simulink model "adcddcxaui_pass15"  (Simulink 6.2)
settings: Solver=ode45  StartTime=0.0  StopTime=100  RelTol=1e-3
undefined symbols (not defined in the file): BitWidth
libraries: xbsIndex_r3 x402, casper_library x31, xps_library x31
(part 1 of 5)
settings Model: LastModifiedBy=lspitler
settings DebuggingCC: SolverPrmCheckMsg=warning

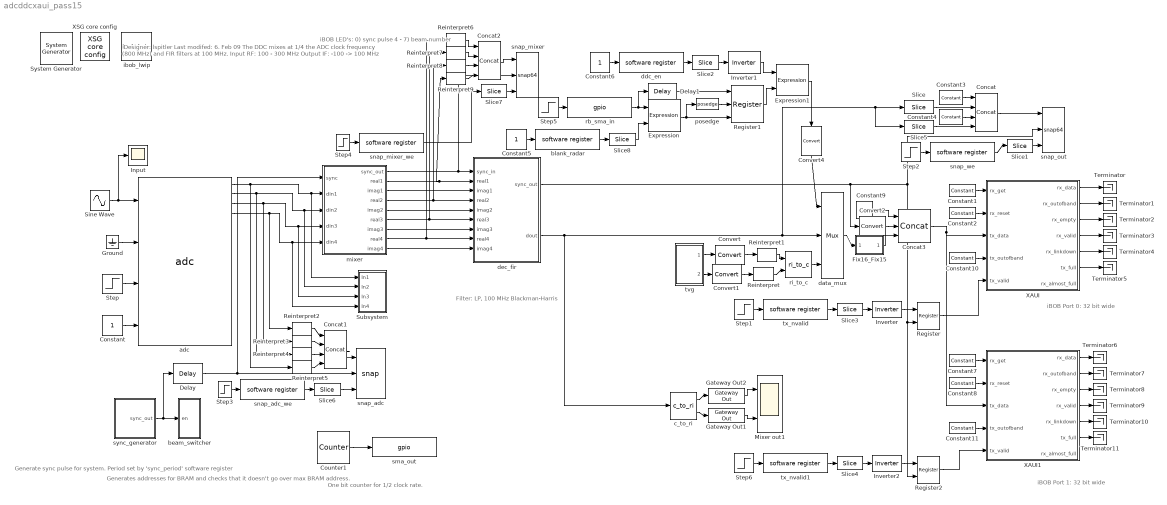
== system adcddcxaui_pass15 ==
  note: Designer: lspitler
      | Last modifed: 6. Feb 09
      | The DDC mixes at 1/4 the ADC clock frequency (800 MHz)
      | and FIR filters at 100 MHz.
      | Input RF: 100 - 300 MHz
      | Output IF: -100 -> 100 MHz
  note: Filter:
      | LP, 100 MHz Blackman-Harris
  note: iBOB Port 0: 32 bit wide
  note: One bit counter
      | for 1/2 clock rate.
  note: Generate sync pulse for system.
      | Period set by 'sync_period'
      | software register
  note: iBOB LED's:
      | 0) sync pulse
      | 4 - 7) beam number
  note: Generates addresses
      | for BRAM and checks
      | that it doesn't go over
      | max BRAM address.
  note: iBOB Port 1: 32 bit wide
  " System Generator" : xbsIndex_r3/ System Generator  Tag=genX  xilinxfamily=Virtex2P  part=xc2vp50  speed=-7  package=ff1152  synthesis_tool=XST  directory=./adcddcxaui_pass/sysgen  testbench=off  simulink_period=1  sysclk_period=5  incr_netlist=off  trim_vbits=Everywhere in SubSystem  dbl_ovrd=According to Block Masks  core_generation=According to Block Masks  run_coregen=off  deprecated_control=off  eval_field=0
      settings: AttributesFormatString=System\nGenerator
  Concat : xbsIndex_r3/Concat  num_inputs=4  explicit_period=on  period=1  dbl_ovrd=off
  Concat1 : xbsIndex_r3/Concat  num_inputs=4  explicit_period=on  period=1  dbl_ovrd=off
  Concat2 : xbsIndex_r3/Concat  num_inputs=4  explicit_period=on  period=1  dbl_ovrd=off
  Concat3 : xbsIndex_r3/Concat  num_inputs=3  explicit_period=on  period=1  dbl_ovrd=off
  Constant : Constant
  Constant1 : xbsIndex_r3/Constant  const=1  equ=P=C  arith_type=Boolean  n_bits=1  bin_pt=0  opselect=C  inp2=PCIN>>17  opr=+  inp1=P  carry=CIN  iostate=0  explicit_period=on  period=1  dbl_ovrd=off
  Constant10 : xbsIndex_r3/Constant  const=0  equ=P=C  arith_type=Unsigned  n_bits=4  bin_pt=0  opselect=C  inp2=PCIN>>17  opr=+  inp1=P  carry=CIN  iostate=0  explicit_period=on  period=1  dbl_ovrd=off
  Constant11 : xbsIndex_r3/Constant  const=0  equ=P=C  arith_type=Unsigned  n_bits=4  bin_pt=0  opselect=C  inp2=PCIN>>17  opr=+  inp1=P  carry=CIN  iostate=0  explicit_period=on  period=1  dbl_ovrd=off
  Constant2 : xbsIndex_r3/Constant  const=0  equ=P=C  arith_type=Boolean  n_bits=1  bin_pt=0  opselect=C  inp2=PCIN>>17  opr=+  inp1=P  carry=CIN  iostate=0  explicit_period=on  period=1  dbl_ovrd=off
  Constant3 : xbsIndex_r3/Constant  const=0  equ=P=C  arith_type=Unsigned  n_bits=16  bin_pt=0  opselect=C  inp2=PCIN>>17  opr=+  inp1=P  carry=CIN  iostate=0  explicit_period=on  period=1  dbl_ovrd=off
  Constant4 : xbsIndex_r3/Constant  const=0  equ=P=C  arith_type=Unsigned  n_bits=16  bin_pt=0  opselect=C  inp2=PCIN>>17  opr=+  inp1=P  carry=CIN  iostate=0  explicit_period=on  period=1  dbl_ovrd=off
  Constant5 : Constant
  Constant6 : Constant
  Constant7 : xbsIndex_r3/Constant  const=1  equ=P=C  arith_type=Boolean  n_bits=1  bin_pt=0  opselect=C  inp2=PCIN>>17  opr=+  inp1=P  carry=CIN  iostate=0  explicit_period=on  period=1  dbl_ovrd=off
  Constant8 : xbsIndex_r3/Constant  const=0  equ=P=C  arith_type=Boolean  n_bits=1  bin_pt=0  opselect=C  inp2=PCIN>>17  opr=+  inp1=P  carry=CIN  iostate=0  explicit_period=on  period=1  dbl_ovrd=off
  Constant9 : xbsIndex_r3/Constant  const=0  equ=P=C  arith_type=Unsigned  n_bits=1  bin_pt=0  opselect=C  inp2=PCIN>>17  opr=+  inp1=P  carry=CIN  iostate=0  explicit_period=on  period=1  dbl_ovrd=off
  Convert : xbsIndex_r3/Convert  arith_type=Unsigned  n_bits=16  bin_pt=0  quantization=Truncate  overflow=Wrap  latency=0  explicit_period=on  period=1  dbl_ovrd=off  show_param=off  inserted_by_tool=off  pipeline=off
      settings: xl_area=[0, 0, 0, 0, 0, 0, 0]
  Convert1 : xbsIndex_r3/Convert  arith_type=Unsigned  n_bits=16  bin_pt=0  quantization=Truncate  overflow=Wrap  latency=0  explicit_period=on  period=1  dbl_ovrd=off  show_param=off  inserted_by_tool=off  pipeline=off
      settings: xl_area=[0, 0, 0, 0, 0, 0, 0]
  Convert2 : xbsIndex_r3/Convert  arith_type=Unsigned  n_bits=1  bin_pt=0  quantization=Truncate  overflow=Wrap  latency=1  explicit_period=on  period=1  dbl_ovrd=off  show_param=off  inserted_by_tool=off  pipeline=off
      settings: xl_area=[0, 0, 0, 0, 0, 0, 0]
  Convert4 : xbsIndex_r3/Convert  Orientation=down  arith_type=Unsigned  n_bits=1  bin_pt=0  quantization=Truncate  overflow=Wrap  latency=0  explicit_period=on  period=1  dbl_ovrd=off  show_param=off  inserted_by_tool=off  pipeline=off
      settings: xl_area=[0, 0, 0, 0, 0, 0, 0]
  Counter1 : xbsIndex_r3/Counter  cnt_type=Free Running  n_bits=1  bin_pt=0  arith_type=Unsigned  start_count=0  cnt_to=Inf  cnt_by_val=1  operation=Up  explicit_period=off  period=1  load_pin=off  rst=off  en=off  dbl_ovrd=off  show_param=off  use_rpm=on  gen_core=off
      settings: xl_area=[0, 0, 0, 0, 0, 0, 0]
  Delay : xbsIndex_r3/Delay  latency=8  reg_retiming=off  explicit_period=on  period=1  en=off  accept_only_valid=off  init_zero=on  dbl_ovrd=off  show_param=off
      settings: xl_area=[0, 0, 0, 0, 0, 0, 0]
  Delay1 : xbsIndex_r3/Delay  latency=1  reg_retiming=off  explicit_period=on  period=1  en=off  accept_only_valid=off  init_zero=on  dbl_ovrd=off  show_param=off
      settings: xl_area=[0, 0, 0, 0, 0, 0, 0]
  Expression : xbsIndex_r3/Expression  expression=a & b  precision=Full  arith_type=Unsigned  n_bits=8  bin_pt=2  align_bp=on  latency=1  explicit_period=on  period=1  en=off  dbl_ovrd=off  show_param=off
      settings: xl_area=[0, 0, 0, 0, 0, 0, 0]
  Expression1 : xbsIndex_r3/Expression  expression=a | b  precision=Full  arith_type=Unsigned  n_bits=8  bin_pt=2  align_bp=on  latency=0  explicit_period=on  period=1  en=off  dbl_ovrd=off  show_param=off
      settings: xl_area=[0, 0, 0, 0, 0, 0, 0]
  Fix16_Fix15 : Subsystem
  Gateway Out1 : xbsIndex_r3/Gateway Out  output_type=Double  nbits=8  bin_pt=6  arith_type=Boolean  quantization=Truncate  overflow=Wrap  hdl_port=on  timing_constraint=None  locs_specified=off  LOCs={}  needs_fixed_name=off  show_param=off
      settings: xl_area=[0, 0, 0, 0, 0, 0, 0]
  Gateway Out2 : xbsIndex_r3/Gateway Out  output_type=Double  nbits=8  bin_pt=6  arith_type=Boolean  quantization=Truncate  overflow=Wrap  hdl_port=on  timing_constraint=None  locs_specified=off  LOCs={}  needs_fixed_name=off  show_param=off
      settings: xl_area=[0, 0, 0, 0, 0, 0, 0]
  Ground : Ground
  Input : Scope
      settings: SaveName=ScopeData2
  Inverter : xbsIndex_r3/Inverter  latency=0  explicit_period=on  period=1  en=off  dbl_ovrd=off  show_param=off
      settings: xl_area=[0, 0, 0, 0, 0, 0, 0]
  Inverter1 : xbsIndex_r3/Inverter  latency=0  explicit_period=off  period=1  en=off  dbl_ovrd=off  show_param=off
      settings: xl_area=[0, 0, 0, 0, 0, 0, 0]
  Inverter2 : xbsIndex_r3/Inverter  latency=0  explicit_period=on  period=1  en=off  dbl_ovrd=off  show_param=off
      settings: xl_area=[0, 0, 0, 0, 0, 0, 0]
  Mixer out1 : Scope  NumInputPorts=2
      settings: YMin=-5~-5  YMax=5~5
  Register : xbsIndex_r3/Register  init=0  reg_only_valid=off  explicit_period=on  period=1  rst=off  en=on  out_en=off  dbl_ovrd=off  show_param=off
      settings: xl_area=[0, 0, 0, 0, 0, 0, 0]
  Register1 : xbsIndex_r3/Register  init=0  reg_only_valid=off  explicit_period=on  period=1  rst=on  en=on  out_en=off  dbl_ovrd=off  show_param=off
      settings: xl_area=[0, 0, 0, 0, 0, 0, 0]
  Register2 : xbsIndex_r3/Register  init=0  reg_only_valid=off  explicit_period=on  period=1  rst=off  en=on  out_en=off  dbl_ovrd=off  show_param=off
      settings: xl_area=[0, 0, 0, 0, 0, 0, 0]
  Reinterpret : xbsIndex_r3/Reinterpret  force_arith_type=on  arith_type="Signed  (2's comp)"  force_bin_pt=on  bin_pt=15  force_valid=on
  Reinterpret1 : xbsIndex_r3/Reinterpret  force_arith_type=on  arith_type="Signed  (2's comp)"  force_bin_pt=on  bin_pt=15  force_valid=on
  Reinterpret{2..9} (8 alike) : xbsIndex_r3/Reinterpret  force_arith_type=on  arith_type=Unsigned  force_bin_pt=on  bin_pt=0  force_valid=on
  Sine Wave : Sin  Amplitude=0.95  Frequency=2*3.1415*(11/8)  Samples=4  SampleTime=0.25  Offset=1
  Slice : xbsIndex_r3/Slice  mode=Upper Bit Location + Width  nbits=16  bit1=0  base1=MSB of Input  bit0=0  base0=LSB of Input  boolean_output=off  explicit_period=on  period=1  dbl_ovrd=off
  Slice{1..4,6..8} (7 alike) : xbsIndex_r3/Slice  mode=Lower Bit Location + Width  nbits=1  bit1=0  base1=MSB of Input  bit0=0  base0=LSB of Input  boolean_output=on  explicit_period=off  period=1  dbl_ovrd=off
  Slice5 : xbsIndex_r3/Slice  mode=Lower Bit Location + Width  nbits=16  bit1=0  base1=MSB of Input  bit0=0  base0=LSB of Input  boolean_output=off  explicit_period=on  period=1  dbl_ovrd=off
  Step{,1..6} (7 alike) : Step  SampleTime=0
  Subsystem : Subsystem
  Terminator{,1..11} (12 alike) : Terminator
  XAUI : Subsystem  Tag=xps:xaui  AncestorBlock=xps_library/XAUI  mask(xaui){demux=2, port=iBOB:0, show_param=off, pre_emph=3, swing=800}
      mask prompts: show_param "---------------------- Show Implementation Parameters -----------------------------------------------------------------------------------"; pre_emph "Pre-emphasis"; swing "Differential swing"
      mask help: XAUI block for sending and receiving point-to-point, streaming data over the BEE2 and iBOB's CX4 connectors. NOTE: A new version of this block is in development.
      mask init:
      | xaui_mask;
      mask Help: eval('xlWeb([getenv(''MLIB_ROOT''), ''\doc\html\com_xaui\com_xaui.html''])')
      mask StyleString: popup(1|2),popup(iBOB:0|iBOB:1|BEE2_ctrl:0|BEE2_ctrl:1|BEE2_usr:0|BEE2_usr:1|BEE2_usr:2|BEE2_usr:3|CORR:0),checkbox,popup(0|1|2|3),popup(400|500|600|700|800)
      mask CallbackString:
      | ||myname=gcb;
      | if strcmp(get_param(myname, 'show_param'), 'on')
      |     set_param(myname, 'MaskVisibilities', {'on','on','on','on','on'});
      | else
      |     set_param(myname, 'MaskVisibilities', {'on','on','on','off','off'});
      | end||
  XAUI1 : Subsystem  Tag=xps:xaui  AncestorBlock=xps_library/XAUI  mask(xaui){demux=2, port=iBOB:1, show_param=off, pre_emph=3, swing=800}
      mask prompts: show_param "---------------------- Show Implementation Parameters -----------------------------------------------------------------------------------"; pre_emph "Pre-emphasis"; swing "Differential swing"
      mask help: XAUI block for sending and receiving point-to-point, streaming data over the BEE2 and iBOB's CX4 connectors. NOTE: A new version of this block is in development.
      mask init:
      | xaui_mask;
      mask Help: eval('xlWeb([getenv(''MLIB_ROOT''), ''\doc\html\com_xaui\com_xaui.html''])')
      mask StyleString: popup(1|2),popup(iBOB:0|iBOB:1|BEE2_ctrl:0|BEE2_ctrl:1|BEE2_usr:0|BEE2_usr:1|BEE2_usr:2|BEE2_usr:3|CORR:0),checkbox,popup(0|1|2|3),popup(400|500|600|700|800)
      mask CallbackString:
      | ||myname=gcb;
      | if strcmp(get_param(myname, 'show_param'), 'on')
      |     set_param(myname, 'MaskVisibilities', {'on','on','on','on','on'});
      | else
      |     set_param(myname, 'MaskVisibilities', {'on','on','on','off','off'});
      | end||
  XSG core config : xps_library/XSG core config  Tag=xps:xsg  hw_sys=iBOB  ibob_linux=off  clk_src=adc0_clk  gpio_clk_io_group=iBOB:sma  gpio_clk_bit_index=0  clk_rate=200  sample_period=1  synthesis_tool=XST  mpc_type=powerpc405
  adc : xps_library/adc  Tag=xps:adc  adc_brd=iBOB:adc0  adc_clk_rate=800  adc_interleave=off  sample_period=1
  beam_switcher : Subsystem
  blank_radar : xps_library/software register  Tag=xps:sw_reg  io_dir=From Processor  arith_type=Unsigned  bitwidth=32  bin_pt=0  sample_period=1  gw_name=adcddcxaui_pass15_blank_radar_user_data_out
  c_to_ri : casper_library/Misc/c_to_ri  n_bits=16  bin_pt=15
      settings: AttributesFormatString=16_15 r/i
  data_mux : xbsIndex_r3/Mux  inputs=2  precision=Full  arith_type="Signed  (2's comp)"  n_bits=8  bin_pt=2  quantization=Truncate  overflow=Wrap  latency=1  explicit_period=on  period=1  en=off  dbl_ovrd=off  show_param=off  mux_type=off  use_rpm=off  gen_core=off
      settings: xl_area=[0, 0, 0, 0, 0, 0, 0]
  ddc_en : xps_library/software register  Tag=xps:sw_reg  io_dir=From Processor  arith_type=Unsigned  bitwidth=32  bin_pt=0  sample_period=1  gw_name=adcddcxaui_pass15_ddc_en_user_data_out
  dec_fir : Subsystem  AncestorBlock=casper_library/Downconverter/dec_fir  mask(dec_fir){n_inputs=4, coeff=[-2.32022704382012e-007 -1.96793901412143e-006 -6.75154059522534e-006 -6.84714551426329e-006 1.40951673085967e-005 6.32691079378998e-005 0.00010979324523175 7.49325945610502e-005 -0.000118431156085725 -0.000436437229681919 -0.000646606487019754 -0.00038661995841418 0.000545438664656682 0.00182028229313871 0.00247093665916482 0.00136692957063967 -0.00179924993407727 -0.00564405140037139 -0.00725034616519259 -0.00381996817794863 0.0048188087277704 0.014580065732477 0.0181905286238286 0.00938133540413822 -0.0116934149100173 -0.0353791342600711 -0.0448597099993105 -0.0240746309704666 0.0324249154639043 0.113465227678761 0.193526756592295 0.243273145290241 0.243273145290241 0.193526756592295 0.113465227678761 0.0324249154639043 -0.0240746309704666 -0.0448597099993105 -0.0353791342600711 -0.0116934149100173 0.00938133540413823 0.0181905286238286 0.014580065732477 0.0048188087277704 -0.00381996817794864 -0.00725034616519259 -0.00564405140037139 -0.00179924993407727 0.00136692957063967 0.00247093665916482 0.00182028229313871 0.000545438664656683 -0.00038661995841418 -0.000646606487019753 -0.00043643722968192 -0.000118431156085725 7.49325945610503e-005 0.00010979324523175 6.32691079379003e-005 1.40951673085965e-005 -6.84714551426338e-006 -6.75154059522503e-006 -1.96793901412178e-006 -2.32022704382012e-007], n_bits=16, quantization=Truncate, add_latency=2, mult_latency=2}
      mask prompts: n_inputs "Number of Parallel Streams"; coeff "Coefficients"; n_bits "Bit Width Out"; quantization "Quantization Behavior"; add_latency "Add Latency"; mult_latency "Mult Latency"
      mask help: FIR filter which can handle multiple time samples in parallel and decimates down to 1 time sample. If coefficients are symmetric, will automatically fold before multiplying.
      mask init:
      | dec_fir_init(gcb, ...
      |     'n_inputs', n_inputs, ...
      |     'coeff', coeff, ...
      |     'n_bits', n_bits, ...
      |     'quantization', quantization, ...
      |     'add_latency', add_latency, ...
      |     'mult_latency', mult_latency);
      settings: AttributesFormatString=|
      | 64 taps
      | 16_15 r/i
      mask Help:
      | <h1>Description</h1>
      | 
      | FIR filter which can handle multiple time samples in parallel and decimates down to 1 time sample.  If coefficients are symmetric, will automatically fold before multiplying.
      | 
      | <h2>Mask Parameters</h2>
      | 
      | <b>Number of Parallel Streams</b> (n_inputs): The number of time samples which arrive in parallel.<br><br>
      | 
      | <b>Coefficients</b> (coeff): The FIR coefficients.  If this vector is symmetric, the FIR will automatically fold before multiplying.<br><br>
      | 
      | <b>Bit Width Out</b> (n_bits): The number of bits in each real/imag sample of the complex number that is output.<br><br>
      | 
      | <b>Quantization Behavior</b> (quantization): The quantization behavior used in converting to the output bit width.<br><br>
      | 
      | 
      | <b>Add Latency</b> (add_latency) = The latency of adders/converters.<br><br>
      | 
      | <b>Mult Latency</b> (mult_latency) = The latency of multipliers.<br><br>
      mask StyleString: edit,edit,edit,popup(Truncate|Round  (unbiased: +/- Inf)|Round  (unbiased: Even Values)),edit,edit
  ibob_lwip : xps_library/ibob_lwip
  mixer : Subsystem  AncestorBlock=casper_library/Downconverter/mixer  mask(mixer){freq_div=4, freq=1, nstreams=4, n_bits=8, bram_latency=2, mult_latency=3}
      mask prompts: freq_div "Frequency Divisions (M)"; freq "Mixing Frequency (? / M*2pi)"; nstreams "Number of Parallel Streams"; n_bits "Bit Width"; bram_latency "BRAM Latency"; mult_latency "Mult Latency"
      mask help: Digitally mixes an input signal (which can be several samples in parallel) with an LO of the indicated frequency (which is some fraction of the native FPGA clock rate).
      mask init:
      | mixer_init(gcb, ...
      |     'freq_div', freq_div, ...
      |     'freq', freq, ...
      |     'nstreams', nstreams, ...
      |     'n_bits', n_bits, ...
      |     'bram_latency', bram_latency, ...
      |     'mult_latency', mult_latency);
      settings: AttributesFormatString=lo at -1/4
      mask Help:
      | <h1>Description</h1>
      | 
      | Digitally mixes an input signal (which can be several samples in parallel) with an LO of the indicated frequency (which is some fraction of the native FPGA clock rate).
      | 
      | <h2>Mask Parameters</h2>
      | 
      | <b>Frequency Divisions</b> (freq_div):  The (power of 2) denominator of the mixing frequency. <br><br>
      | 
      | <b>Mixing Frequency</b> (freq) = The numerator of the mixing frequency.<br><br>
      | 
      | <b>Number of Parallel Streams</b> (nstreams) = The number of samples which arrive in parallel.<br><br>
      | 
      | <b>Bit Width</b> (n_bits) = The bitwidth of LO samples.<br><br>
      | 
      | <b>BRAM Latency</b> (bram_latency) = The latency of sine/cos lookup table.<br><br>
      | 
      | <b>MULT Latency</b> (mult_latency) = The latency of mixing multipliers.<br><br>
      | 
      | <h2> Usage </h2>
      | M = Frequency Divisions<br>
      | F = Mixing Frequency<br>
      | M and F must both be integers, and M must be a power of 2. The ratio F/M should equal the ratio f/r where r is the data rate of the sampled signal. For example, an F/M of 3/16 would downmix an 800Msps signal with an LO of 150MHz.
  posedge : casper_library/Misc/posedge  Tag=Rising Edge Detector
  rb_sma_in : xps_library/gpio  Tag=xps:gpio  io_group=iBOB:sma  io_dir=in  arith_type=Boolean  bitwidth=1  bin_pt=0  bit_index=1  sample_period=1  use_single_ended=off  use_ddr=off  reg_iob=on  reg_clk_phase=0  termination=None
  ri_to_c : casper_library/Misc/ri_to_c
  sma_out : xps_library/gpio  Tag=xps:gpio  io_group=iBOB:sma  io_dir=out  arith_type=Boolean  bitwidth=1  bin_pt=0  bit_index=0  sample_period=1  use_single_ended=off  use_ddr=off  reg_iob=on  reg_clk_phase=0  termination=None
  snap_adc : casper_library/Scopes/snap  nsamples=11
  snap_adc_we : xps_library/software register  Tag=xps:sw_reg  io_dir=From Processor  arith_type=Unsigned  bitwidth=32  bin_pt=0  sample_period=1  gw_name=adcddcxaui_pass15_snap_adc_we_user_data_out
  snap_mixer : casper_library/Scopes/snap64  nsamples=11
  snap_mixer_we : xps_library/software register  Tag=xps:sw_reg  io_dir=From Processor  arith_type=Unsigned  bitwidth=32  bin_pt=0  sample_period=1  gw_name=adcddcxaui_pass15_snap_mixer_we_user_data_out
  snap_out : casper_library/Scopes/snap64  nsamples=11
  snap_we : xps_library/software register  Tag=xps:sw_reg  io_dir=From Processor  arith_type=Unsigned  bitwidth=32  bin_pt=0  sample_period=1  gw_name=adcddcxaui_pass15_snap_we_user_data_out
  sync_generator : Subsystem
  tvg : Subsystem
  tx_nvalid : xps_library/software register  Tag=xps:sw_reg  io_dir=From Processor  arith_type=Unsigned  bitwidth=32  bin_pt=0  sample_period=1  gw_name=adcddcxaui_pass15_tx_nvalid_user_data_out
  tx_nvalid1 : xps_library/software register  Tag=xps:sw_reg  io_dir=From Processor  arith_type=Unsigned  bitwidth=32  bin_pt=0  sample_period=1  gw_name=adcddcxaui_pass15_tx_nvalid1_user_data_out
  wires:
  mixer/1(sync_out) -> dec_fir/1(sync_in), snap_mixer/2
  mixer/2(real1) -> dec_fir/2(real1), Reinterpret9/1
  mixer/3(imag1) -> dec_fir/3(imag1)
  mixer/4(real2) -> dec_fir/4(real2), Reinterpret8/1
  mixer/5(imag2) -> dec_fir/5(imag2)
  mixer/6(real3) -> dec_fir/6(real3), Reinterpret7/1
  mixer/7(imag3) -> dec_fir/7(imag3)
  mixer/8(real4) -> dec_fir/8(real4), Reinterpret6/1
  mixer/9(imag4) -> dec_fir/9(imag4)
  dec_fir/2(dout) -> c_to_ri/1, data_mux/2, Slice/1, Slice5/1
  Constant1/1 -> XAUI/1(rx_get)
  Sine Wave/1 -> adc/1, Input/1
  Ground/1 -> adc/2
  adc/1 -> mixer/2(din1), Subsystem/1(In1), Reinterpret5/1
  adc/2 -> mixer/3(din2), Subsystem/2(In2), Reinterpret4/1
  adc/3 -> mixer/4(din3), Subsystem/3(In3), Reinterpret3/1
  adc/4 -> mixer/5(din4), Subsystem/4(In4), Reinterpret2/1
  Step/1 -> adc/3
  Constant/1 -> adc/4
  dec_fir/1(sync_out) -> snap_out/2, Register/2, Register2/2, Convert2/1
  snap_we/1 -> Slice1/1
  Step2/1 -> snap_we/1
  Slice1/1 -> snap_out/3
  XAUI/1(rx_data) -> Terminator/1
  XAUI/2(rx_outofband) -> Terminator1/1
  XAUI/3(rx_empty) -> Terminator2/1
  XAUI/4(rx_valid) -> Terminator3/1
  XAUI/5(rx_linkdown) -> Terminator4/1
  XAUI/6(tx_full) -> Terminator5/1
  Step1/1 -> tx_nvalid/1
  tx_nvalid/1 -> Slice3/1
  Inverter/1 -> Register/1
  Slice3/1 -> Inverter/1
  Register/1 -> XAUI/5(tx_valid)
  Expression1/1 -> Convert4/1
  tvg/1(re_out) -> Convert/1
  tvg/2(im_out) -> Convert1/1
  Convert/1 -> Reinterpret1/1
  Convert1/1 -> Reinterpret/1
  ri_to_c/1 -> data_mux/3
  Reinterpret1/1 -> ri_to_c/1
  Reinterpret/1 -> ri_to_c/2
  Counter1/1 -> sma_out/1
  sync_generator/1(sync_out) -> beam_switcher/1(en), Delay/1
  Delay/1 -> snap_adc/2, mixer/1(sync)
  Concat/1 -> snap_out/1
  Constant3/1 -> Concat/1
  Slice/1 -> Concat/2
  Constant4/1 -> Concat/3
  Slice5/1 -> Concat/4
  Reinterpret2/1 -> Concat1/1
  snap_adc_we/1 -> Slice6/1
  Step3/1 -> snap_adc_we/1
  Slice6/1 -> snap_adc/3
  Concat1/1 -> snap_adc/1
  Reinterpret3/1 -> Concat1/2
  Reinterpret4/1 -> Concat1/3
  Reinterpret5/1 -> Concat1/4
  snap_mixer_we/1 -> Slice7/1
  Step4/1 -> snap_mixer_we/1
  Slice7/1 -> snap_mixer/3
  Reinterpret6/1 -> Concat2/1
  Reinterpret7/1 -> Concat2/2
  Reinterpret8/1 -> Concat2/3
  Reinterpret9/1 -> Concat2/4
  Concat2/1 -> snap_mixer/1
  c_to_ri/2 -> Gateway Out1/1
  Gateway Out1/1 -> Mixer out1/2
  c_to_ri/1 -> Gateway Out2/1
  Gateway Out2/1 -> Mixer out1/1
  rb_sma_in/1 -> Expression/1, Delay1/1
  blank_radar/1 -> Slice8/1
  Slice8/1 -> Expression/2
  Constant5/1 -> blank_radar/1
  Step5/1 -> rb_sma_in/1
  Expression/1 -> Register1/3, posedge/1
  posedge/1 -> Register1/2
  Register1/1 -> Expression1/2
  Constant6/1 -> ddc_en/1
  ddc_en/1 -> Slice2/1
  Inverter1/1 -> Expression1/1
  Delay1/1 -> Register1/1
  Constant2/1 -> XAUI/2(rx_reset)
  Slice2/1 -> Inverter1/1
  Constant7/1 -> XAUI1/1(rx_get)
  Constant8/1 -> XAUI1/2(rx_reset)
  Step6/1 -> tx_nvalid1/1
  tx_nvalid1/1 -> Slice4/1
  Inverter2/1 -> Register2/1
  Slice4/1 -> Inverter2/1
  Register2/1 -> XAUI1/5(tx_valid)
  XAUI1/1(rx_data) -> Terminator6/1
  XAUI1/2(rx_outofband) -> Terminator7/1
  XAUI1/3(rx_empty) -> Terminator8/1
  XAUI1/4(rx_valid) -> Terminator9/1
  XAUI1/5(rx_linkdown) -> Terminator10/1
  XAUI1/6(tx_full) -> Terminator11/1
  Convert4/1 -> data_mux/1
  data_mux/1 -> Fix16_Fix15/1(In1)
  Constant9/1 -> Concat3/1
  Concat3/1 -> XAUI/3(tx_data), XAUI1/3(tx_data)
  Constant10/1 -> XAUI/4(tx_outofband)
  Constant11/1 -> XAUI1/4(tx_outofband)
  Fix16_Fix15/1(Out1) -> Concat3/3
  Convert2/1 -> Concat3/2

== system adcddcxaui_pass15/Fix16_Fix15 ==
  In1 : Inport  Port=1  LatchInput=off
  Convert5 : xbsIndex_r3/Convert  arith_type="Signed  (2's comp)"  n_bits=15  bin_pt=14  quantization=Truncate  overflow=Wrap  latency=0  explicit_period=on  period=1  dbl_ovrd=off  show_param=off  inserted_by_tool=off  pipeline=off
      settings: xl_area=[0, 0, 0, 0, 0, 0, 0]
  Convert6 : xbsIndex_r3/Convert  arith_type="Signed  (2's comp)"  n_bits=15  bin_pt=14  quantization=Truncate  overflow=Wrap  latency=0  explicit_period=on  period=1  dbl_ovrd=off  show_param=off  inserted_by_tool=off  pipeline=off
      settings: xl_area=[0, 0, 0, 0, 0, 0, 0]
  c_to_ri1 : casper_library/Misc/c_to_ri  n_bits=16  bin_pt=15
      settings: AttributesFormatString=16_15 r/i
  ri_to_c1 : casper_library/Misc/ri_to_c
  Out1 : Outport
  wires:
  c_to_ri1/1 -> Convert5/1
  c_to_ri1/2 -> Convert6/1
  Convert5/1 -> ri_to_c1/1
  Convert6/1 -> ri_to_c1/2
  In1/1 -> c_to_ri1/1
  ri_to_c1/1 -> Out1/1

== system adcddcxaui_pass15/Subsystem ==
  In1 : Inport  Port=1  LatchInput=off
  In2 : Inport  Port=2  LatchInput=off
  In3 : Inport  Port=3  LatchInput=off
  In4 : Inport  Port=4  LatchInput=off
  ADC out : Scope  NumInputPorts=4
      settings: YMin=-5~-5~-5~-5  YMax=5~5~5~5  SaveName=ScopeData3
  Gateway Out{2..5} (4 alike) : xbsIndex_r3/Gateway Out  output_type=Double  nbits=8  bin_pt=6  arith_type=Boolean  quantization=Truncate  overflow=Wrap  hdl_port=on  timing_constraint=None  locs_specified=off  LOCs={}  needs_fixed_name=off  show_param=off
      settings: xl_area=[0, 0, 0, 0, 0, 0, 0]
  wires:
  Gateway Out2/1 -> ADC out/1
  Gateway Out3/1 -> ADC out/2
  Gateway Out4/1 -> ADC out/3
  Gateway Out5/1 -> ADC out/4
  In1/1 -> Gateway Out2/1
  In2/1 -> Gateway Out3/1
  In3/1 -> Gateway Out4/1
  In4/1 -> Gateway Out5/1

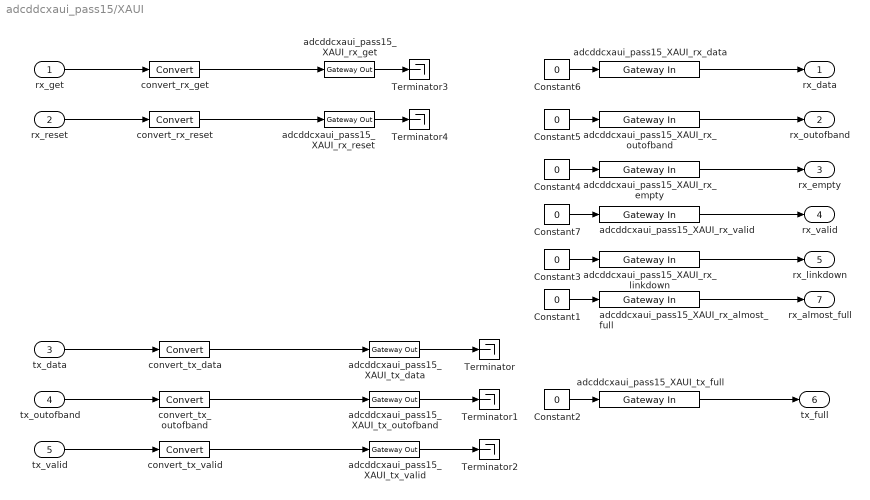
== system adcddcxaui_pass15/XAUI ==
  rx_get : Inport  Port=1  LatchInput=off
  rx_reset : Inport  Port=2  LatchInput=off
  tx_data : Inport  Port=3  LatchInput=off
  tx_outofband : Inport  Port=4  LatchInput=off
  tx_valid : Inport  Port=5  LatchInput=off
  Constant{1..7} (7 alike) : Constant  Value=0
  Terminator{,1..4} (5 alike) : Terminator
  adcddcxaui_pass15_XAUI_rx_almost_full : xbsIndex_r3/Gateway In  arith_type=Boolean  n_bits=1  bin_pt=0  quantization=Truncate  overflow=Wrap  period=1  timing_constraint=None  locs_specified=off  LOCs={}  needs_fixed_name=off  dbl_ovrd=off  show_param=off
      settings: xl_area=[0, 0, 0, 0, 0, 0, 0]
  adcddcxaui_pass15_XAUI_rx_data : xbsIndex_r3/Gateway In  arith_type=Unsigned  n_bits=32  bin_pt=0  quantization=Truncate  overflow=Wrap  period=1  timing_constraint=None  locs_specified=off  LOCs={}  needs_fixed_name=off  dbl_ovrd=off  show_param=off
      settings: xl_area=[0, 0, 0, 0, 0, 0, 0]
  adcddcxaui_pass15_XAUI_rx_empty : xbsIndex_r3/Gateway In  arith_type=Boolean  n_bits=1  bin_pt=0  quantization=Truncate  overflow=Wrap  period=1  timing_constraint=None  locs_specified=off  LOCs={}  needs_fixed_name=off  dbl_ovrd=off  show_param=off
      settings: xl_area=[0, 0, 0, 0, 0, 0, 0]
  adcddcxaui_pass15_XAUI_rx_get : xbsIndex_r3/Gateway Out  output_type=Double  nbits=8  bin_pt=6  arith_type=Boolean  quantization=Truncate  overflow=Wrap  hdl_port=on  timing_constraint=None  locs_specified=off  LOCs={}  needs_fixed_name=off  show_param=off
      settings: xl_area=[0, 0, 0, 0, 0, 0, 0]
  adcddcxaui_pass15_XAUI_rx_linkdown : xbsIndex_r3/Gateway In  arith_type=Boolean  n_bits=1  bin_pt=0  quantization=Truncate  overflow=Wrap  period=1  timing_constraint=None  locs_specified=off  LOCs={}  needs_fixed_name=off  dbl_ovrd=off  show_param=off
      settings: xl_area=[0, 0, 0, 0, 0, 0, 0]
  adcddcxaui_pass15_XAUI_rx_outofband : xbsIndex_r3/Gateway In  arith_type=Unsigned  n_bits=4  bin_pt=0  quantization=Truncate  overflow=Wrap  period=1  timing_constraint=None  locs_specified=off  LOCs={}  needs_fixed_name=off  dbl_ovrd=off  show_param=off
      settings: xl_area=[0, 0, 0, 0, 0, 0, 0]
  adcddcxaui_pass15_XAUI_rx_reset : xbsIndex_r3/Gateway Out  output_type=Double  nbits=8  bin_pt=6  arith_type=Boolean  quantization=Truncate  overflow=Wrap  hdl_port=on  timing_constraint=None  locs_specified=off  LOCs={}  needs_fixed_name=off  show_param=off
      settings: xl_area=[0, 0, 0, 0, 0, 0, 0]
  adcddcxaui_pass15_XAUI_rx_valid : xbsIndex_r3/Gateway In  arith_type=Boolean  n_bits=1  bin_pt=0  quantization=Truncate  overflow=Wrap  period=1  timing_constraint=None  locs_specified=off  LOCs={}  needs_fixed_name=off  dbl_ovrd=off  show_param=off
      settings: xl_area=[0, 0, 0, 0, 0, 0, 0]
  adcddcxaui_pass15_XAUI_tx_data : xbsIndex_r3/Gateway Out  output_type=Double  nbits=8  bin_pt=6  arith_type=Boolean  quantization=Truncate  overflow=Wrap  hdl_port=on  timing_constraint=None  locs_specified=off  LOCs={}  needs_fixed_name=off  show_param=off
      settings: xl_area=[0, 0, 0, 0, 0, 0, 0]
  adcddcxaui_pass15_XAUI_tx_full : xbsIndex_r3/Gateway In  arith_type=Boolean  n_bits=1  bin_pt=0  quantization=Truncate  overflow=Wrap  period=1  timing_constraint=None  locs_specified=off  LOCs={}  needs_fixed_name=off  dbl_ovrd=off  show_param=off
      settings: xl_area=[0, 0, 0, 0, 0, 0, 0]
  adcddcxaui_pass15_XAUI_tx_outofband : xbsIndex_r3/Gateway Out  output_type=Double  nbits=8  bin_pt=6  arith_type=Boolean  quantization=Truncate  overflow=Wrap  hdl_port=on  timing_constraint=None  locs_specified=off  LOCs={}  needs_fixed_name=off  show_param=off
      settings: xl_area=[0, 0, 0, 0, 0, 0, 0]
  adcddcxaui_pass15_XAUI_tx_valid : xbsIndex_r3/Gateway Out  output_type=Double  nbits=8  bin_pt=6  arith_type=Boolean  quantization=Truncate  overflow=Wrap  hdl_port=on  timing_constraint=None  locs_specified=off  LOCs={}  needs_fixed_name=off  show_param=off
      settings: xl_area=[0, 0, 0, 0, 0, 0, 0]
  convert_rx_get : xbsIndex_r3/Convert  arith_type=Boolean  n_bits=64  bin_pt=0  quantization=Truncate  overflow=Wrap  latency=0  explicit_period=off  period=1  dbl_ovrd=off  show_param=off  inserted_by_tool=off  pipeline=off
      settings: xl_area=[0, 0, 0, 0, 0, 0, 0]
  convert_rx_reset : xbsIndex_r3/Convert  arith_type=Boolean  n_bits=1  bin_pt=0  quantization=Truncate  overflow=Wrap  latency=0  explicit_period=off  period=1  dbl_ovrd=off  show_param=off  inserted_by_tool=off  pipeline=off
      settings: xl_area=[0, 0, 0, 0, 0, 0, 0]
  convert_tx_data : xbsIndex_r3/Convert  arith_type=Unsigned  n_bits=32  bin_pt=0  quantization=Truncate  overflow=Wrap  latency=0  explicit_period=off  period=1  dbl_ovrd=off  show_param=off  inserted_by_tool=off  pipeline=off
      settings: xl_area=[0, 0, 0, 0, 0, 0, 0]
  convert_tx_outofband : xbsIndex_r3/Convert  arith_type=Unsigned  n_bits=4  bin_pt=0  quantization=Truncate  overflow=Wrap  latency=0  explicit_period=off  period=1  dbl_ovrd=off  show_param=off  inserted_by_tool=off  pipeline=off
      settings: xl_area=[0, 0, 0, 0, 0, 0, 0]
  convert_tx_valid : xbsIndex_r3/Convert  arith_type=Boolean  n_bits=1  bin_pt=0  quantization=Truncate  overflow=Wrap  latency=0  explicit_period=off  period=1  dbl_ovrd=off  show_param=off  inserted_by_tool=off  pipeline=off
      settings: xl_area=[0, 0, 0, 0, 0, 0, 0]
  rx_data : Outport
  rx_outofband : Outport  Port=2
  rx_empty : Outport  Port=3
  rx_valid : Outport  Port=4
  rx_linkdown : Outport  Port=5
  tx_full : Outport  Port=6
  rx_almost_full : Outport  Port=7
  wires:
  Constant1/1 -> adcddcxaui_pass15_XAUI_rx_almost_full/1
  adcddcxaui_pass15_XAUI_rx_almost_full/1 -> rx_almost_full/1
  adcddcxaui_pass15_XAUI_rx_valid/1 -> rx_valid/1
  Constant7/1 -> adcddcxaui_pass15_XAUI_rx_valid/1
  adcddcxaui_pass15_XAUI_rx_reset/1 -> Terminator4/1
  adcddcxaui_pass15_XAUI_rx_get/1 -> Terminator3/1
  Constant6/1 -> adcddcxaui_pass15_XAUI_rx_data/1
  Constant5/1 -> adcddcxaui_pass15_XAUI_rx_outofband/1
  Constant4/1 -> adcddcxaui_pass15_XAUI_rx_empty/1
  Constant3/1 -> adcddcxaui_pass15_XAUI_rx_linkdown/1
  Constant2/1 -> adcddcxaui_pass15_XAUI_tx_full/1
  adcddcxaui_pass15_XAUI_tx_valid/1 -> Terminator2/1
  adcddcxaui_pass15_XAUI_tx_outofband/1 -> Terminator1/1
  adcddcxaui_pass15_XAUI_tx_data/1 -> Terminator/1
  adcddcxaui_pass15_XAUI_tx_full/1 -> tx_full/1
  convert_tx_valid/1 -> adcddcxaui_pass15_XAUI_tx_valid/1
  tx_valid/1 -> convert_tx_valid/1
  convert_tx_outofband/1 -> adcddcxaui_pass15_XAUI_tx_outofband/1
  tx_outofband/1 -> convert_tx_outofband/1
  convert_tx_data/1 -> adcddcxaui_pass15_XAUI_tx_data/1
  tx_data/1 -> convert_tx_data/1
  adcddcxaui_pass15_XAUI_rx_linkdown/1 -> rx_linkdown/1
  adcddcxaui_pass15_XAUI_rx_empty/1 -> rx_empty/1
  adcddcxaui_pass15_XAUI_rx_outofband/1 -> rx_outofband/1
  adcddcxaui_pass15_XAUI_rx_data/1 -> rx_data/1
  convert_rx_reset/1 -> adcddcxaui_pass15_XAUI_rx_reset/1
  rx_reset/1 -> convert_rx_reset/1
  convert_rx_get/1 -> adcddcxaui_pass15_XAUI_rx_get/1
  rx_get/1 -> convert_rx_get/1

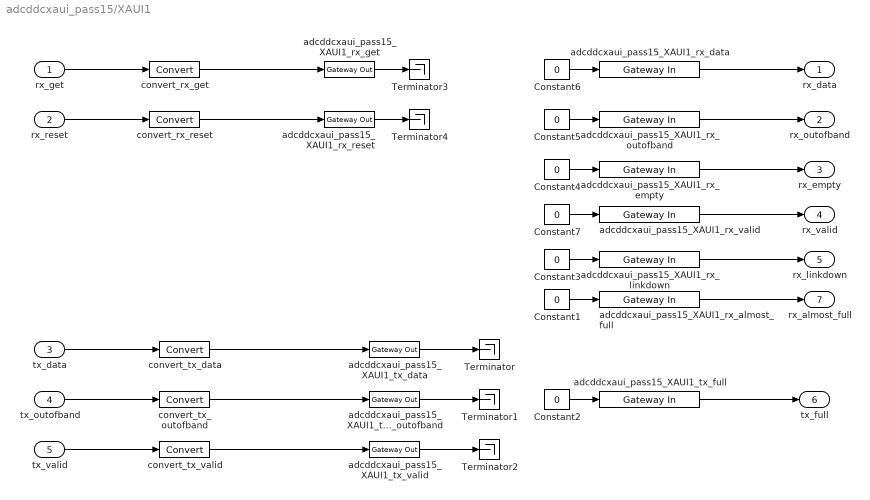
== system adcddcxaui_pass15/XAUI1 ==
  rx_get : Inport  Port=1  LatchInput=off
  rx_reset : Inport  Port=2  LatchInput=off
  tx_data : Inport  Port=3  LatchInput=off
  tx_outofband : Inport  Port=4  LatchInput=off
  tx_valid : Inport  Port=5  LatchInput=off
  Constant{1..7} (7 alike) : Constant  Value=0
  Terminator{,1..4} (5 alike) : Terminator
  adcddcxaui_pass15_XAUI1_rx_almost_full : xbsIndex_r3/Gateway In  arith_type=Boolean  n_bits=1  bin_pt=0  quantization=Truncate  overflow=Wrap  period=1  timing_constraint=None  locs_specified=off  LOCs={}  needs_fixed_name=off  dbl_ovrd=off  show_param=off
      settings: xl_area=[0, 0, 0, 0, 0, 0, 0]
  adcddcxaui_pass15_XAUI1_rx_data : xbsIndex_r3/Gateway In  arith_type=Unsigned  n_bits=32  bin_pt=0  quantization=Truncate  overflow=Wrap  period=1  timing_constraint=None  locs_specified=off  LOCs={}  needs_fixed_name=off  dbl_ovrd=off  show_param=off
      settings: xl_area=[0, 0, 0, 0, 0, 0, 0]
  adcddcxaui_pass15_XAUI1_rx_empty : xbsIndex_r3/Gateway In  arith_type=Boolean  n_bits=1  bin_pt=0  quantization=Truncate  overflow=Wrap  period=1  timing_constraint=None  locs_specified=off  LOCs={}  needs_fixed_name=off  dbl_ovrd=off  show_param=off
      settings: xl_area=[0, 0, 0, 0, 0, 0, 0]
  adcddcxaui_pass15_XAUI1_rx_get : xbsIndex_r3/Gateway Out  output_type=Double  nbits=8  bin_pt=6  arith_type=Boolean  quantization=Truncate  overflow=Wrap  hdl_port=on  timing_constraint=None  locs_specified=off  LOCs={}  needs_fixed_name=off  show_param=off
      settings: xl_area=[0, 0, 0, 0, 0, 0, 0]
  adcddcxaui_pass15_XAUI1_rx_linkdown : xbsIndex_r3/Gateway In  arith_type=Boolean  n_bits=1  bin_pt=0  quantization=Truncate  overflow=Wrap  period=1  timing_constraint=None  locs_specified=off  LOCs={}  needs_fixed_name=off  dbl_ovrd=off  show_param=off
      settings: xl_area=[0, 0, 0, 0, 0, 0, 0]
  adcddcxaui_pass15_XAUI1_rx_outofband : xbsIndex_r3/Gateway In  arith_type=Unsigned  n_bits=4  bin_pt=0  quantization=Truncate  overflow=Wrap  period=1  timing_constraint=None  locs_specified=off  LOCs={}  needs_fixed_name=off  dbl_ovrd=off  show_param=off
      settings: xl_area=[0, 0, 0, 0, 0, 0, 0]
  adcddcxaui_pass15_XAUI1_rx_reset : xbsIndex_r3/Gateway Out  output_type=Double  nbits=8  bin_pt=6  arith_type=Boolean  quantization=Truncate  overflow=Wrap  hdl_port=on  timing_constraint=None  locs_specified=off  LOCs={}  needs_fixed_name=off  show_param=off
      settings: xl_area=[0, 0, 0, 0, 0, 0, 0]
  adcddcxaui_pass15_XAUI1_rx_valid : xbsIndex_r3/Gateway In  arith_type=Boolean  n_bits=1  bin_pt=0  quantization=Truncate  overflow=Wrap  period=1  timing_constraint=None  locs_specified=off  LOCs={}  needs_fixed_name=off  dbl_ovrd=off  show_param=off
      settings: xl_area=[0, 0, 0, 0, 0, 0, 0]
  adcddcxaui_pass15_XAUI1_tx_data : xbsIndex_r3/Gateway Out  output_type=Double  nbits=8  bin_pt=6  arith_type=Boolean  quantization=Truncate  overflow=Wrap  hdl_port=on  timing_constraint=None  locs_specified=off  LOCs={}  needs_fixed_name=off  show_param=off
      settings: xl_area=[0, 0, 0, 0, 0, 0, 0]
  adcddcxaui_pass15_XAUI1_tx_full : xbsIndex_r3/Gateway In  arith_type=Boolean  n_bits=1  bin_pt=0  quantization=Truncate  overflow=Wrap  period=1  timing_constraint=None  locs_specified=off  LOCs={}  needs_fixed_name=off  dbl_ovrd=off  show_param=off
      settings: xl_area=[0, 0, 0, 0, 0, 0, 0]
  adcddcxaui_pass15_XAUI1_tx_outofband : xbsIndex_r3/Gateway Out  output_type=Double  nbits=8  bin_pt=6  arith_type=Boolean  quantization=Truncate  overflow=Wrap  hdl_port=on  timing_constraint=None  locs_specified=off  LOCs={}  needs_fixed_name=off  show_param=off
      settings: xl_area=[0, 0, 0, 0, 0, 0, 0]
  adcddcxaui_pass15_XAUI1_tx_valid : xbsIndex_r3/Gateway Out  output_type=Double  nbits=8  bin_pt=6  arith_type=Boolean  quantization=Truncate  overflow=Wrap  hdl_port=on  timing_constraint=None  locs_specified=off  LOCs={}  needs_fixed_name=off  show_param=off
      settings: xl_area=[0, 0, 0, 0, 0, 0, 0]
  convert_rx_get : xbsIndex_r3/Convert  arith_type=Boolean  n_bits=64  bin_pt=0  quantization=Truncate  overflow=Wrap  latency=0  explicit_period=off  period=1  dbl_ovrd=off  show_param=off  inserted_by_tool=off  pipeline=off
      settings: xl_area=[0, 0, 0, 0, 0, 0, 0]
  convert_rx_reset : xbsIndex_r3/Convert  arith_type=Boolean  n_bits=1  bin_pt=0  quantization=Truncate  overflow=Wrap  latency=0  explicit_period=off  period=1  dbl_ovrd=off  show_param=off  inserted_by_tool=off  pipeline=off
      settings: xl_area=[0, 0, 0, 0, 0, 0, 0]
  convert_tx_data : xbsIndex_r3/Convert  arith_type=Unsigned  n_bits=32  bin_pt=0  quantization=Truncate  overflow=Wrap  latency=0  explicit_period=off  period=1  dbl_ovrd=off  show_param=off  inserted_by_tool=off  pipeline=off
      settings: xl_area=[0, 0, 0, 0, 0, 0, 0]
  convert_tx_outofband : xbsIndex_r3/Convert  arith_type=Unsigned  n_bits=4  bin_pt=0  quantization=Truncate  overflow=Wrap  latency=0  explicit_period=off  period=1  dbl_ovrd=off  show_param=off  inserted_by_tool=off  pipeline=off
      settings: xl_area=[0, 0, 0, 0, 0, 0, 0]
  convert_tx_valid : xbsIndex_r3/Convert  arith_type=Boolean  n_bits=1  bin_pt=0  quantization=Truncate  overflow=Wrap  latency=0  explicit_period=off  period=1  dbl_ovrd=off  show_param=off  inserted_by_tool=off  pipeline=off
      settings: xl_area=[0, 0, 0, 0, 0, 0, 0]
  rx_data : Outport
  rx_outofband : Outport  Port=2
  rx_empty : Outport  Port=3
  rx_valid : Outport  Port=4
  rx_linkdown : Outport  Port=5
  tx_full : Outport  Port=6
  rx_almost_full : Outport  Port=7
  wires:
  rx_get/1 -> convert_rx_get/1
  convert_rx_get/1 -> adcddcxaui_pass15_XAUI1_rx_get/1
  rx_reset/1 -> convert_rx_reset/1
  convert_rx_reset/1 -> adcddcxaui_pass15_XAUI1_rx_reset/1
  adcddcxaui_pass15_XAUI1_rx_data/1 -> rx_data/1
  adcddcxaui_pass15_XAUI1_rx_outofband/1 -> rx_outofband/1
  adcddcxaui_pass15_XAUI1_rx_empty/1 -> rx_empty/1
  adcddcxaui_pass15_XAUI1_rx_linkdown/1 -> rx_linkdown/1
  tx_data/1 -> convert_tx_data/1
  convert_tx_data/1 -> adcddcxaui_pass15_XAUI1_tx_data/1
  tx_outofband/1 -> convert_tx_outofband/1
  convert_tx_outofband/1 -> adcddcxaui_pass15_XAUI1_tx_outofband/1
  tx_valid/1 -> convert_tx_valid/1
  convert_tx_valid/1 -> adcddcxaui_pass15_XAUI1_tx_valid/1
  adcddcxaui_pass15_XAUI1_tx_full/1 -> tx_full/1
  adcddcxaui_pass15_XAUI1_tx_data/1 -> Terminator/1
  adcddcxaui_pass15_XAUI1_tx_outofband/1 -> Terminator1/1
  adcddcxaui_pass15_XAUI1_tx_valid/1 -> Terminator2/1
  Constant2/1 -> adcddcxaui_pass15_XAUI1_tx_full/1
  Constant3/1 -> adcddcxaui_pass15_XAUI1_rx_linkdown/1
  Constant4/1 -> adcddcxaui_pass15_XAUI1_rx_empty/1
  Constant5/1 -> adcddcxaui_pass15_XAUI1_rx_outofband/1
  Constant6/1 -> adcddcxaui_pass15_XAUI1_rx_data/1
  adcddcxaui_pass15_XAUI1_rx_get/1 -> Terminator3/1
  adcddcxaui_pass15_XAUI1_rx_reset/1 -> Terminator4/1
  Constant7/1 -> adcddcxaui_pass15_XAUI1_rx_valid/1
  adcddcxaui_pass15_XAUI1_rx_valid/1 -> rx_valid/1
  adcddcxaui_pass15_XAUI1_rx_almost_full/1 -> rx_almost_full/1
  Constant1/1 -> adcddcxaui_pass15_XAUI1_rx_almost_full/1

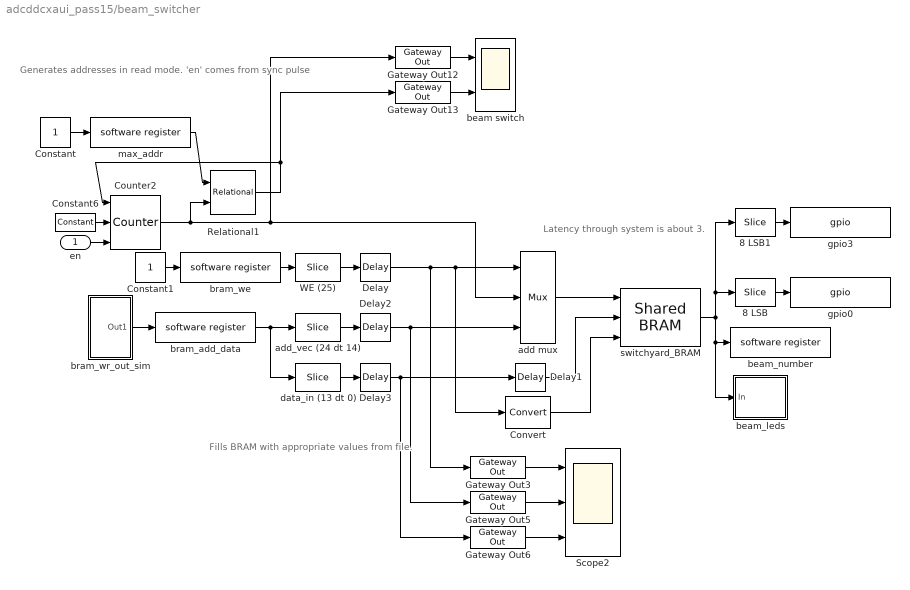
== system adcddcxaui_pass15/beam_switcher ==
  note: Generates addresses
      | in read mode.
      | 'en' comes from sync
      | pulse
  note: Fills BRAM with
      | appropriate values
      | from file.
  note: Latency through
      | system is about 3.
  en : Inport  Port=1  LatchInput=off
  8 LSB : xbsIndex_r3/Slice  mode=Lower Bit Location + Width  nbits=8  bit1=10  base1=MSB of Input  bit0=0  base0=LSB of Input  boolean_output=off  explicit_period=on  period=1  dbl_ovrd=off
  8 LSB1 : xbsIndex_r3/Slice  mode=Lower Bit Location + Width  nbits=8  bit1=10  base1=MSB of Input  bit0=0  base0=LSB of Input  boolean_output=off  explicit_period=on  period=1  dbl_ovrd=off
  Constant : Constant
  Constant1 : Constant
  Constant6 : xbsIndex_r3/Constant  const=0  equ=P=C  arith_type=Unsigned  n_bits=32  bin_pt=0  opselect=C  inp2=PCIN>>17  opr=+  inp1=P  carry=CIN  iostate=0  explicit_period=on  period=1  dbl_ovrd=off
  Convert : xbsIndex_r3/Convert  arith_type=Boolean  n_bits=8  bin_pt=6  quantization=Truncate  overflow=Wrap  latency=1  explicit_period=on  period=1  dbl_ovrd=off  show_param=off  inserted_by_tool=off  pipeline=off
      settings: xl_area=[0, 0, 0, 0, 0, 0, 0]
  Counter2 : xbsIndex_r3/Counter  cnt_type=Free Running  n_bits=32  bin_pt=0  arith_type=Unsigned  start_count=0  cnt_to=Inf  cnt_by_val=1  operation=Up  explicit_period=on  period=1  load_pin=on  rst=off  en=on  dbl_ovrd=off  show_param=off  use_rpm=on  gen_core=off
      settings: xl_area=[0, 0, 0, 0, 0, 0, 0]
  Delay{,1..3} (4 alike) : xbsIndex_r3/Delay  latency=1  reg_retiming=off  explicit_period=on  period=1  en=off  accept_only_valid=off  init_zero=on  dbl_ovrd=off  show_param=off
      settings: xl_area=[0, 0, 0, 0, 0, 0, 0]
  Gateway Out{3,5..6,12..13} (5 alike) : xbsIndex_r3/Gateway Out  output_type=Double  nbits=8  bin_pt=6  arith_type=Boolean  quantization=Truncate  overflow=Wrap  hdl_port=on  timing_constraint=None  locs_specified=off  LOCs={}  needs_fixed_name=off  show_param=off
      settings: xl_area=[0, 0, 0, 0, 0, 0, 0]
  Relational1 : xbsIndex_r3/Relational  mode=a=b  latency=1  explicit_period=on  period=1  en=off  dbl_ovrd=off  show_param=off
      settings: xl_area=[0, 0, 0, 0, 0, 0, 0]
  Scope2 : Scope  NumInputPorts=3
      settings: YMin=-5~-5~-5  YMax=5~5~5  SaveName=ScopeData8
  WE (25) : xbsIndex_r3/Slice  mode=Lower Bit Location + Width  nbits=1  bit1=10  base1=MSB of Input  bit0=0  base0=LSB of Input  boolean_output=off  explicit_period=on  period=1  dbl_ovrd=off
  add mux : xbsIndex_r3/Mux  inputs=2  precision=Full  arith_type="Signed  (2's comp)"  n_bits=8  bin_pt=2  quantization=Truncate  overflow=Wrap  latency=1  explicit_period=on  period=1  en=off  dbl_ovrd=off  show_param=off  mux_type=off  use_rpm=off  gen_core=off
      settings: xl_area=[0, 0, 0, 0, 0, 0, 0]
  "add_vec (24 dt 14) " : xbsIndex_r3/Slice  mode=Lower Bit Location + Width  nbits=11  bit1=0  base1=MSB of Input  bit0=14  base0=LSB of Input  boolean_output=off  explicit_period=on  period=1  dbl_ovrd=off
  beam switch : Scope  NumInputPorts=2
      settings: YMin=-5~-5  YMax=5~5  SaveName=ScopeData6
  beam_leds : Subsystem
  beam_number : xps_library/software register  Tag=xps:sw_reg  io_dir=To Processor  arith_type=Unsigned  bitwidth=32  bin_pt=0  sample_period=1  gw_name=adcddcxaui_pass15_beam_switcher_beam_number_user_data_in
  bram_add_data : xps_library/software register  Tag=xps:sw_reg  io_dir=From Processor  arith_type=Unsigned  bitwidth=32  bin_pt=0  sample_period=1  gw_name=adcddcxaui_pass15_beam_switcher_bram_add_data_user_data_out
  bram_we : xps_library/software register  Tag=xps:sw_reg  io_dir=From Processor  arith_type=Unsigned  bitwidth=32  bin_pt=0  sample_period=1  gw_name=adcddcxaui_pass15_beam_switcher_bram_we_user_data_out
  bram_wr_out_sim : Subsystem  mask{we_enable=0, ram_sel=3, add_vec=512, data_in=32}
      mask prompts: we_enable "Write enable"; ram_sel "RAM selector (1 = Re; 2 = Im; 3 = both)"; add_vec "RAM address"; data_in "Data in"
  data_in (13 dt 0) : xbsIndex_r3/Slice  mode=Lower Bit Location + Width  nbits=14  bit1=0  base1=MSB of Input  bit0=0  base0=LSB of Input  boolean_output=off  explicit_period=on  period=1  dbl_ovrd=off
  gpio0 : xps_library/gpio  Tag=xps:gpio  io_group=iBOB:gpio0  io_dir=out  arith_type=Unsigned  bitwidth=8  bin_pt=0  bit_index=[0:7]  sample_period=1  use_single_ended=off  use_ddr=off  reg_iob=on  reg_clk_phase=0  termination=None
  gpio3 : xps_library/gpio  Tag=xps:gpio  io_group=iBOB:gpio3  io_dir=out  arith_type=Unsigned  bitwidth=8  bin_pt=0  bit_index=[0:7]  sample_period=1  use_single_ended=off  use_ddr=off  reg_iob=on  reg_clk_phase=0  termination=None
  max_addr : xps_library/software register  Tag=xps:sw_reg  io_dir=From Processor  arith_type=Unsigned  bitwidth=32  bin_pt=0  sample_period=1  gw_name=adcddcxaui_pass15_beam_switcher_max_addr_user_data_out
  switchyard_BRAM : xps_library/Shared BRAM  Tag=xps:bram  arith_type=Unsigned  addr_width=11  data_width=32  data_bin_pt=0  init_vals=[0:2^11-1]  sample_rate=1
  wires:
  Counter2/1 -> Relational1/2, add mux/2, Gateway Out12/1
  Relational1/1 -> Counter2/1, Gateway Out13/1
  switchyard_BRAM/1 -> beam_number/1, beam_leds/1(In), 8 LSB/1, 8 LSB1/1
  Constant6/1 -> Counter2/2
  en/1 -> Counter2/3
  Gateway Out12/1 -> beam switch/1
  Gateway Out13/1 -> beam switch/2
  Delay3/1 -> Delay1/1, Gateway Out6/1
  Delay2/1 -> add mux/3, Gateway Out5/1
  Delay/1 -> Gateway Out3/1, add mux/1, Convert/1
  bram_wr_out_sim/1(Out1) -> bram_add_data/1
  data_in (13 dt 0)/1 -> Delay3/1
  "add_vec (24 dt 14) "/1 -> Delay2/1
  bram_add_data/1 -> data_in (13 dt 0)/1, "add_vec (24 dt 14) "/1
  Gateway Out3/1 -> Scope2/1
  WE (25)/1 -> Delay/1
  add mux/1 -> switchyard_BRAM/1
  Convert/1 -> switchyard_BRAM/3
  Delay1/1 -> switchyard_BRAM/2
  Gateway Out5/1 -> Scope2/2
  Gateway Out6/1 -> Scope2/3
  max_addr/1 -> Relational1/1
  Constant/1 -> max_addr/1
  bram_we/1 -> WE (25)/1
  Constant1/1 -> bram_we/1
  8 LSB/1 -> gpio0/1
  8 LSB1/1 -> gpio3/1
